simulink model "simulink_model"  (R2017a)
settings: Solver=VariableStepAuto  StartTime=0.0  StopTime=.1  MaxStep=1e-4  RelTol=1e-3
libraries: powerlib x33
settings Model: Creator=platinum  LastModifiedBy=platinum

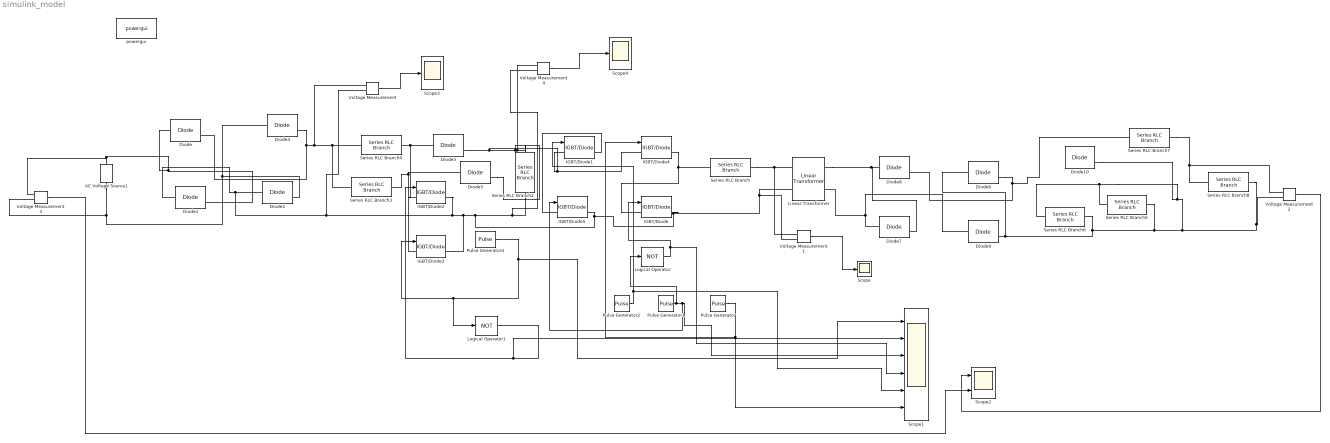
== system simulink_model ==
  AC Voltage Source1 : powerlib/Electrical Sources/AC Voltage Source  Amplitude=240  Phase=0  Frequency=50  SampleTime=0  Measurements=None  BusType=swing  Pref=10e3  Qref=0  Qmin=-inf  Qmax=+inf
  Diode{,1..10} (11 alike) : powerlib/Power Electronics/Diode  Ron=0.001  Lon=0  Vf=0.8  IC=0  UseSnubber=0  Rs=500  Cs=250e-9  Measurements=on
  IGBT/Diode{,1,4..5} (4 alike) : powerlib/Power Electronics/IGBT//Diode  Ron=1e-3  Rs=1e5  Cs=45e-13  Measurements=on
  IGBT/Diode2 : powerlib/Power Electronics/IGBT//Diode  Ron=1e-3  Rs=99e-4  Cs=inf  Measurements=on
  IGBT/Diode3 : powerlib/Power Electronics/IGBT//Diode  Ron=1e-3  Rs=99e-4  Cs=inf  Measurements=on
  Linear Transformer : powerlib/Elements/Linear Transformer  UNITS=SI  NominalPower=[ 3e3 50 ]  winding1=[300 1e-3 0]  winding2="[400  1e-3 0]"  ThreeWindings=off  winding3=[3.15e+05 7.8765e+11 2.2168e+08]  RmLm=[ 1 2e-6 ]  Measurements=None  DataType=on
  Logical Operator : Logic  Operator=NOT  Inputs=1  AllPortsSameDT=off  OutDataTypeStr=boolean
  Logical Operator1 : Logic  Operator=NOT  Inputs=1  AllPortsSameDT=off  OutDataTypeStr=boolean
  Pulse Generator : DiscretePulseGenerator  PulseType=Time based  Period=.00001  PulseWidth=20  PhaseDelay=.0000035
  Pulse Generator1 : DiscretePulseGenerator  PulseType=Time based  Period=.00001  PulseWidth=50  PhaseDelay=00
  Pulse Generator2 : DiscretePulseGenerator  PulseType=Time based  Period=.00001  PulseWidth=50
  Pulse Generator4 : DiscretePulseGenerator  PulseType=Time based  Period=.000014  PulseWidth=50
  Scope : Scope
  Scope1 : Scope  NumInputPorts=6
  Scope2 : Scope  NumInputPorts=2
  Scope3 : Scope
  Scope4 : Scope
  Series RLC Branch : powerlib/Elements/Series RLC Branch  LConnTagsString=__new0  RConnTagsString=__new0  BranchType=L  Resistance=1  Inductance=8e-7  SetiL0=on  InitialCurrent=8e-7  Capacitance=1e-6  Setx0=off  InitialVoltage=0  Measurements=None
  Series RLC Branch2 : powerlib/Elements/Series RLC Branch  LConnTagsString=__new0  RConnTagsString=__new0  BranchType=C  Resistance=1  Inductance=1e-3  SetiL0=off  InitialCurrent=0  Capacitance=33e-6  Setx0=on  InitialVoltage=400  Measurements=None
  Series RLC Branch3 : powerlib/Elements/Series RLC Branch  LConnTagsString=__new0  RConnTagsString=__new0  BranchType=L  Resistance=1  Inductance=4e-4  SetiL0=off  InitialCurrent=0  Capacitance=1e-6  Setx0=off  InitialVoltage=0  Measurements=None
  Series RLC Branch4 : powerlib/Elements/Series RLC Branch  LConnTagsString=__new0  RConnTagsString=__new0  BranchType=L  Resistance=1  Inductance=4e-4  SetiL0=off  InitialCurrent=0  Capacitance=1e-6  Setx0=off  InitialVoltage=0  Measurements=None
  Series RLC Branch5 : powerlib/Elements/Series RLC Branch  LConnTagsString=__new0  RConnTagsString=__new0  BranchType=C  Resistance=1  Inductance=1e-3  SetiL0=off  InitialCurrent=0  Capacitance=33e-6  Setx0=on  InitialVoltage=33e-6  Measurements=None
  Series RLC Branch6 : powerlib/Elements/Series RLC Branch  LConnTagsString=__new0  RConnTagsString=__new0  BranchType=R  Resistance=100  Inductance=1e-3  SetiL0=off  InitialCurrent=0  Capacitance=1e-6  Setx0=off  InitialVoltage=0  Measurements=None
  Series RLC Branch7 : powerlib/Elements/Series RLC Branch  LConnTagsString=__new0  RConnTagsString=__new0  BranchType=L  Resistance=1  Inductance=16e-3  SetiL0=off  InitialCurrent=0  Capacitance=1e-6  Setx0=off  InitialVoltage=0  Measurements=None
  Series RLC Branch8 : powerlib/Elements/Series RLC Branch  LConnTagsString=__new0  RConnTagsString=__new0  BranchType=C  Resistance=1  Inductance=1e-3  SetiL0=off  InitialCurrent=0  Capacitance=33e-6  Setx0=on  InitialVoltage=200  Measurements=None
  Voltage Measurement{,1..4} (5 alike) : powerlib/Measurements/Voltage Measurement  PhasorSimulation=off  OutputType=Complex  PSBequivalent=0
  powergui : powerlib/powergui  Priority=1  SimulationMode=Continuous  SampleTime=50e-6  frequency=60  Iterations=50  frequencyindice=0  Pbase=100e6  ErrMax=1e-4  UnitsV=kV  UnitsW=MW  buscounter=0  FunctionMessages=off  echomessages=off  EnableUseOfTLC=off  CurrentSourceSwitches=off  DisableSnubberDevices=off  DisableRonSwitches=off  DisableVfSwitches=off  DisplayEquations=off  SolverType=Tustin/Backward Euler (TBE)  Interpol=off  ExternalGateDelay=off  methode=off  Ts=100  x0status=blocks  SPID=on  SwTol=0  HookPort=off  RestoreLinks=warning  ResistiveCurrentMeasurement=off  Frange=[0:2:500]  Ylog=off  Xlog=on  ShowGrid=off  save=off  variable=ZData  structure=0  ZoomFFT=off  StartTime=0.0  cycles=1  DisplayStyle=1  fundamental=60  FreqAxis=off  MaxFrequency=1000  frequencyindicesteady=1  RmsSteady=1  display=off
  wires:
  Pulse Generator2/1 -> Scope1/5, IGBT/Diode1/1
  Pulse Generator1/1 -> Logical Operator/1, IGBT/Diode5/1, Scope1/3
  Pulse Generator4/1 -> Scope1/1, Logical Operator1/1, IGBT/Diode3/1
  Pulse Generator/1 -> Scope1/6, IGBT/Diode4/1
  Voltage Measurement2/1 -> Scope2/1
  Voltage Measurement3/1 -> Scope2/2
  Voltage Measurement/1 -> Scope3/1
  Logical Operator/1 -> Scope1/4, IGBT/Diode/1
  Voltage Measurement1/1 -> Scope/1
  Logical Operator1/1 -> Scope1/2, IGBT/Diode2/1
  Voltage Measurement4/1 -> Scope4/1
  connections:
  Diode/LConn1 -- Voltage Measurement3/LConn1 -- AC Voltage Source1/RConn1 -- Diode1/RConn1
  Diode2/RConn1 -- Diode4/LConn1 -- Voltage Measurement3/LConn2 -- AC Voltage Source1/LConn1
  Diode4/RConn1 -- Series RLC Branch3/LConn1 -- Series RLC Branch4/LConn1 -- Voltage Measurement/LConn1 -- Diode/RConn1
  Diode5/LConn1 -- IGBT/Diode3/LConn1 -- Series RLC Branch3/RConn1
  Diode3/LConn1 -- IGBT/Diode2/LConn1 -- Series RLC Branch4/RConn1
  IGBT/Diode5/LConn1 -- IGBT/Diode1/RConn1
  IGBT/Diode4/RConn1 -- IGBT/Diode/LConn1 -- Series RLC Branch/LConn1
  Diode8/LConn1 -- Linear Transformer/RConn1 -- Diode7/RConn1
  Diode7/LConn1 -- Linear Transformer/RConn2 -- Diode9/LConn1
  Diode9/RConn1 -- Diode10/RConn1 -- Series RLC Branch5/LConn1 -- Series RLC Branch6/LConn1 -- Series RLC Branch8/RConn1 -- Voltage Measurement2/LConn2 -- Series RLC Branch5/RConn1 -- Series RLC Branch6/RConn1 -- Diode6/LConn1
  Diode6/RConn1 -- Series RLC Branch7/LConn1 -- Diode8/RConn1
  Series RLC Branch7/RConn1 -- Voltage Measurement2/LConn1 -- Series RLC Branch8/LConn1
  Series RLC Branch/RConn1 -- Voltage Measurement1/LConn1 -- Linear Transformer/LConn1
  Series RLC Branch2/LConn1 -- Voltage Measurement4/LConn1 -- Diode3/RConn1 -- IGBT/Diode4/LConn1 -- IGBT/Diode1/LConn1 -- Diode5/RConn1
  Voltage Measurement1/LConn2 -- IGBT/Diode2/RConn1 -- Diode1/LConn1 -- Diode2/LConn1 -- Voltage Measurement/LConn2 -- IGBT/Diode3/RConn1 -- Voltage Measurement4/LConn2 -- Series RLC Branch2/RConn1 -- IGBT/Diode5/RConn1 -- IGBT/Diode/RConn1 -- Linear Transformer/LConn2
